simulink subsystem "octocopter_model"  (R2023a)
settings: Solver=VariableStepAuto  StartTime=0.0  StopTime=10.0  RelTol=1e-3
model mask{m=0, l=0, k_T=0, k_M=0, lxx=0, lyy=0, lzz=0, X0=[0 0 0 0 0 0 0 0 0 0 0 0]}
  mask prompts: m "Mass (kg):"; l "Motor Distance (m):"; k_T "Thrust Coefficient:"; k_M "Moment Coefficient:"; lxx "Moment of Inertial x (kgm^2):"; lyy "Moment of Inertial y (kgm^2):"; lzz "Moment of Inertial z (kgm^2):"; X0 "Initial Conditions:"
values from neighbouring files (symbols this model uses):
  k_M = 8e-5    (= 8e-05)    [drone_data.m]
  k_T = 3e-4    (= 0.0003)    [drone_data.m]
  l = 0.22414    [drone_data.m]
  lxx = 3.426e-5    (= 3.426e-05)    [drone_data.m]
  lyy = 2.00298e-3    (= 0.00200298)    [drone_data.m]
  lzz = 2.01834e-3    (= 0.00201834)    [drone_data.m]
  m = 0.7227    [drone_data.m]
  X0 = zeros(12, 1)    [octocopter_model_test_script.m]
undefined symbols (not defined in the file or in its folder): octocopter_kinematics
settings Model: Creator=mluser  LastModifiedBy=mluser

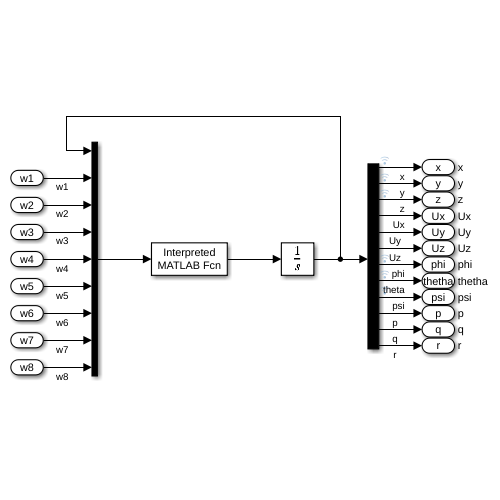
[thumbnail: Simulink's stored preview of the top-level diagram]
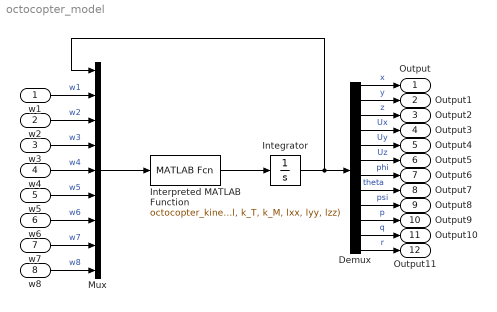
== system octocopter_model ==
  w1 : Inport
  w2 : Inport  Port=2
  w3 : Inport  Port=3
  w4 : Inport  Port=4
  w5 : Inport  Port=5
  w6 : Inport  Port=6
  w7 : Inport  Port=7
  w8 : Inport  Port=8
  Demux : Demux  Outputs=12
  Integrator : Integrator  InitialCondition=X0
  Interpreted MATLAB Function : MATLABFcn  MATLABFcn=octocopter_kinematics(u(1:12), u(13:20), m, l, k_T, k_M, lxx, lyy, lzz)
  Mux : Mux  Inputs=9
  Output : Outport  SignalName=x
  Output1 : Outport  Port=2  SignalName=y
  Output2 : Outport  Port=3  SignalName=z
  Output3 : Outport  Port=4  SignalName=Ux
  Output4 : Outport  Port=5  SignalName=Uy
  Output5 : Outport  Port=6  SignalName=Uz
  Output6 : Outport  Port=7  SignalName=phi
  Output7 : Outport  Port=8  SignalName=thetha
  Output8 : Outport  Port=9  SignalName=psi
  Output9 : Outport  Port=10  SignalName=p
  Output10 : Outport  Port=11  SignalName=q
  Output11 : Outport  Port=12  SignalName=r
  wires:
  Mux/1 -> Interpreted MATLAB Function/1
  Interpreted MATLAB Function/1 -> Integrator/1
  Integrator/1 -> Mux/1, Demux/1
  w1/1 -> Mux/2  "w1"
  Demux/1 -> Output/1  "x"
  Demux/2 -> Output1/1  "y"
  Demux/3 -> Output2/1  "z"
  Demux/7 -> Output6/1  "phi"
  Demux/8 -> Output7/1  "theta"
  Demux/9 -> Output8/1  "psi"
  w2/1 -> Mux/3  "w2"
  w3/1 -> Mux/4  "w3"
  w4/1 -> Mux/5  "w4"
  w5/1 -> Mux/6  "w5"
  w6/1 -> Mux/7  "w6"
  w7/1 -> Mux/8  "w7"
  w8/1 -> Mux/9  "w8"
  Demux/4 -> Output3/1  "Ux"
  Demux/5 -> Output4/1  "Uy"
  Demux/6 -> Output5/1  "Uz"
  Demux/10 -> Output9/1  "p"
  Demux/11 -> Output10/1  "q"
  Demux/12 -> Output11/1  "r"
